simulink model "Case3_IEEE39_UGFLandGFM_2022b"  (R2022b)
settings: Solver=VariableStepAuto  StartTime=0.0  StopTime=30  RelTol=1e-3
InitFcn:
  | IEEE39data_UGFLandGFM;
undefined symbols (not defined in the file): Fref, IBR, line, Sbase, SG, UGFML, Vbase
libraries: spsThreePhaseVIMeasurementLib x66, spsThreePhasePISectionLineLib x35, spsPLL3phLib x25, spsControlledVoltageSourceLib x21, spsThreePhaseParallelRLCLoadLib x21, powerlib_extras x20, spsGroundLib x20, spsMeanLib x20, spsRMSLib x15, spsabctodq0Lib x11, spsThreePhaseSeriesRLCBranchLib x10, slpidlib x10
(part 4 of 5)

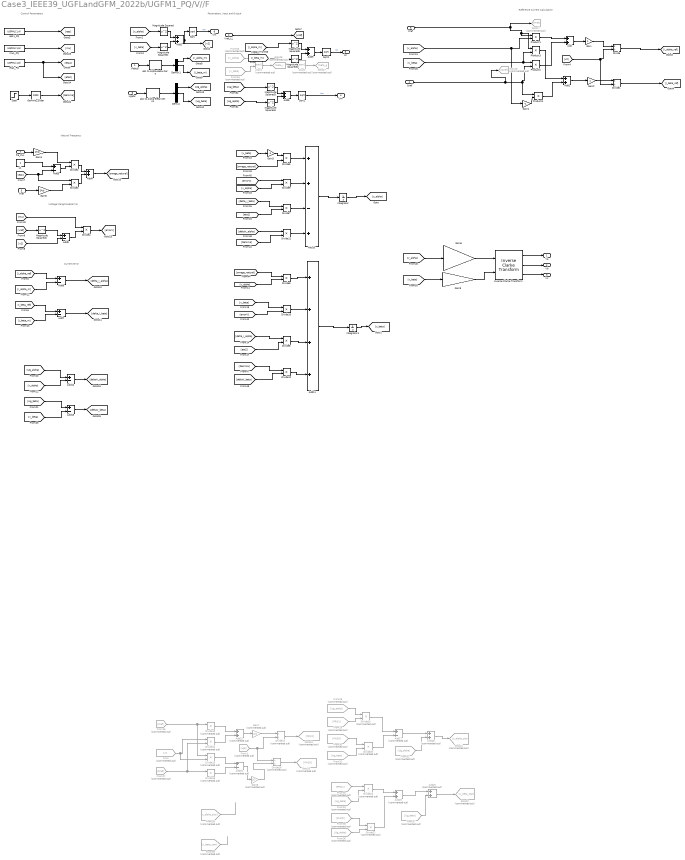
== system Case3_IEEE39_UGFLandGFM_2022b/UGFM1_PQ/V//F ==
  note: Natural Frequency
  note: Voltage Mangnitude Errror
  note: Current Error
  note: Control Parameters
  note: Parameters, Input and Output
  note: Reference Current Calculation
  iFabcb : Inport
  Vref_LL : Inport  Port=2
  Fref : Inport  Port=3
  Qref : Inport  Port=4
  Pref : Inport  Port=5
  Ugabc : Inport  Port=6
  fre_PLL : Inport  Port=7
  Add{,1..2,4,8..9} (6 alike) : Sum
  Add10 : Sum  Inputs=++-+
  Add11 : Sum  Inputs=++++
  Add{3,5..7,12..13} (6 alike) : Sum  Inputs=+-
  Add{15,18..20} (4 alike) : Sum  Commented=on
  Add16 : Sum  Commented=on  Inputs=+-
  Add17 : Sum  Commented=on  Inputs=+-
  Atan1 : Trigonometry  Commented=on  Operator=atan2
  Atan2 : Trigonometry  Commented=on  Operator=atan2
  Demux : Demux  Outputs=3
  Demux1 : Demux  Outputs=3
  Divide : Product  Inputs=*/
  Divide1 : Product  Inputs=*/
  Divide{2..12} (11 alike) : Product  Inputs=**
  Divide{13..16,19..22} (8 alike) : Product  Commented=on  Inputs=**
  Divide17 : Product  Commented=on  Inputs=*/
  Divide18 : Product  Commented=on  Inputs=/*
  From : From  Commented=on  GotoTag=X
  From1 : From  Commented=on  GotoTag=ug2
  From26 : From  Commented=on  GotoTag=Pref
  From27 : From  Commented=on  GotoTag=Qref
  From28 : From  Commented=on  GotoTag=Ug_alpha
  From29 : From  Commented=on  GotoTag=PRQX
  From30 : From  Commented=on  GotoTag=PXQR
  From31 : From  Commented=on  GotoTag=Ug_beta
  From32 : From  Commented=on  GotoTag=Ug_alpha
  From33 : From  Commented=on  GotoTag=PRQX
  From34 : From  Commented=on  GotoTag=Ug_beta
  From35 : From  Commented=on  GotoTag=PXQR
  From36 : From  Commented=on  GotoTag=Ug_alpha
  From37 : From  Commented=on  GotoTag=Ug_beta
  From38 : From  Commented=on  GotoTag=v_alpha_star
  From39 : From  Commented=on  GotoTag=v_beta_star
  From53 : From  Commented=on  GotoTag=v_alpha
  From54 : From  Commented=on  GotoTag=v_beta
  Gain : Gain
  Gain1 : Gain  Gain=-1
  Gain2 : Gain
  Gain3 : Gain  Gain=-1
  Gain4 : Gain  Gain=2*pi
  Gain5 : Gain  Gain=2*pi
  Gain6 : Gain  Gain=Vbase/sqrt(3)*sqrt(2)
  Gain7 : Gain  Commented=on  Gain=2/3
  Gain8 : Gain  Commented=on  Gain=2/3
  Gain9 : Gain  Gain=Vbase/sqrt(3)*sqrt(2)
  Gamma_Slider : simulink/Math Operations/Slider Gain  gain=1000  low=0  high=1000
  Goto17 : Goto  Commented=on  GotoTag=Pref
  Goto18 : Goto  Commented=on  GotoTag=Qref
  Goto19 : Goto  Commented=on  GotoTag=PRQX
  Goto20 : Goto  Commented=on  GotoTag=PXQR
  Goto21 : Goto  Commented=on  GotoTag=v_alpha_star
  Goto22 : Goto  Commented=on  GotoTag=v_beta_star
  Goto27 : Goto  Commented=on  GotoTag=theta_g  TagVisibility=global
  Goto28 : Goto  Commented=on  GotoTag=theta_i  TagVisibility=global
  Integrator : Integrator  InitialCondition=1  LimitOutput=on  UpperSaturationLimit=2  LowerSaturationLimit=-2  ZeroCross=off
  Integrator1 : Integrator  InitialCondition=0.0001  LimitOutput=on  UpperSaturationLimit=2  LowerSaturationLimit=-2  ZeroCross=off
  Inverse Clarke Transform : mcbcontrolslib/Inverse Clarke Transform  PhaseInput=Two inputs  EnPowerInv=off
      settings: LibrarySourceBlock=mcblib/Controls/Math Transforms/Inverse Clarke Transform
  Magnitude Squared{,1..6} (7 alike) : Math  Operator=square
  Product{1..4} (4 alike) : Product
  Sqrt : Sqrt
  Sqrt1 : Sqrt
  Sqrt2 : Sqrt
  Step : Step  Time=0.1  Before=1  After=0  SampleTime=0
  abc to Alpha-Beta-Zero : spsabctoAlphaBetaZeroLib/abc to Alpha-Beta-Zero
  abc to Alpha-Beta-Zero1 : spsabctoAlphaBetaZeroLib/abc to Alpha-Beta-Zero
  eps1_PQ : Constant  Value=UGFML(1,4)
  eta1_PQ : Constant  Value=UGFML(1,6)
  mu1_PQ : Constant  Value=UGFML(1,5)
  u1 : Constant
  Va : Outport
  Vb : Outport  Port=2
  Vc : Outport  Port=3
  Um : Outport  Port=4
  Im : Outport  Port=5
  Vm : Outport  Port=6
  wires:
  iFabcb/1 -> abc to Alpha-Beta-Zero/1
  Inverse Clarke Transform/1 -> Va/1
  Inverse Clarke Transform/2 -> Vb/1
  Inverse Clarke Transform/3 -> Vc/1
  abc to Alpha-Beta-Zero/1 -> Demux1/1
  Integrator1/1 -> [v_beta]
  Pref/1 -> Product3/1, Product1/1, Goto17/1
  [v_alpha] -> Gain1/1, Product1/2
  [v_beta] -> Product3/2, Product2/1
  Qref/1 -> Goto18/1, Product2/2, Product4/1
  Product1/1 -> Add/1
  Product2/1 -> Add/2
  Gain1/1 -> Product4/2
  Product3/1 -> Add1/1
  Product4/1 -> Add1/2
  Add/1 -> Gain/1
  Add1/1 -> Gain2/1
  [v_alpha] -> Magnitude Squared/1
  [v_beta] -> Magnitude Squared1/1
  Magnitude Squared/1 -> Add2/1
  Magnitude Squared1/1 -> Add2/2
  Gain/1 -> Divide/1
  [v2] -> Divide/2, Divide1/2
  Gain2/1 -> Divide1/1
  Divide/1 -> [i_alpha_ref]
  Divide1/1 -> [i_beta_ref]
  u1/1 -> Add3/1
  [eps] -> Divide3/1, Add3/2
  Add3/1 -> Divide2/2
  Fref/1 -> Gain5/1
  Divide2/1 -> Add4/1
  Divide3/1 -> Add4/2
  [v2] -> Add5/2
  Magnitude Squared2/1 -> Add5/1
  Add5/1 -> Divide4/2
  [errorV] -> Divide10/2
  [omega_natural] -> Divide5/2
  [v_beta] -> Gain3/1
  Gain3/1 -> Divide5/1
  [v_alpha] -> Divide6/2
  [i_alpha_ref] -> Add6/1
  [i_alpha_m] -> Add6/2
  [i_beta_ref] -> Add7/1
  Demux1/1 -> [i_alpha_m]
  Demux1/2 -> [i_beta_m]
  [i_beta_m] -> Add7/2
  Add6/1 -> [delta_i_alpha]
  Add7/1 -> [delta_i_beta]
  [delta_i_beta] -> Divide7/1
  [eta1] -> Divide7/2
  Divide7/1 -> Add10/3
  [delta_i_alpha] -> Divide8/1
  [eta2] -> Divide8/2
  Divide8/1 -> Add11/3
  Add10/1 -> Integrator/1
  Add11/1 -> Integrator1/1
  Gain5/1 -> Divide3/2
  Vref_LL/1 -> [vref]
  [vref] -> Magnitude Squared2/1
  [v_alpha] -> Divide9/2
  [v_beta] -> Divide10/1
  Divide5/1 -> Add10/1
  Divide9/1 -> Add10/2
  Divide6/1 -> Add11/1
  Divide10/1 -> Add11/2
  Ugabc/1 -> abc to Alpha-Beta-Zero1/1
  abc to Alpha-Beta-Zero1/1 -> Demux/1
  From38/1 -> ?
  [v_alpha] -> Add12/2
  From39/1 -> ?
  [v_beta] -> Add13/2
  Add12/1 -> [deltaV_alpha]
  Add13/1 -> [deltaV_beta]
  Divide11/1 -> Add10/4
  Divide12/1 -> Add11/4
  eta1_PQ/1 -> [eta2], [eta1]
  Gain4/1 -> Divide2/1
  Demux/1 -> [Ug_alpha]
  Demux/2 -> [Ug_beta]
  From26/1 -> Divide15/1, Divide13/1
  From/1 -> Divide15/2, Divide14/1
  From27/1 -> Divide16/1, Divide14/2
  Divide13/1 -> Add15/1
  Divide14/1 -> Add15/2
  Divide15/1 -> Add16/1
  Divide16/1 -> Add16/2
  Gain7/1 -> Divide17/1
  Gain8/1 -> Divide18/2
  From1/1 -> Divide18/1, Divide17/2
  Add15/1 -> Gain7/1
  Add16/1 -> Gain8/1
  Divide17/1 -> Goto19/1
  Divide18/1 -> Goto20/1
  From28/1 -> Divide19/1
  From29/1 -> Divide19/2
  From30/1 -> Divide20/1
  From31/1 -> Divide20/2
  Divide19/1 -> Add17/1
  Divide20/1 -> Add17/2
  Add17/1 -> Add18/1
  From32/1 -> Add18/2
  From33/1 -> Divide21/1
  From34/1 -> Divide21/2
  From35/1 -> Divide22/1
  From36/1 -> Divide22/2
  Divide21/1 -> Add19/1
  Divide22/1 -> Add19/2
  Add19/1 -> Add20/1
  From37/1 -> Add20/2
  Add18/1 -> Goto21/1
  Add20/1 -> Goto22/1
  [Ug_alpha] -> Add12/1
  [Ug_beta] -> Add13/1
  [mu] -> Divide4/1
  eps1_PQ/1 -> [eps]
  Step/1 -> Gamma_Slider/1
  Gamma_Slider/1 -> [Gamma]
  [Gamma] -> Divide11/2
  Divide4/1 -> [errorV]
  Add4/1 -> [omega_natural]
  [omega_natural] -> Divide6/1
  [errorV] -> Divide9/1
  Integrator/1 -> [v_alpha]
  [v_alpha] -> Gain6/1
  [Gamma] -> Divide12/1
  [deltaV_alpha] -> Divide11/1
  [deltaV_beta] -> Divide12/2
  [v_beta] -> Gain9/1
  Gain6/1 -> Inverse Clarke Transform/1
  Gain9/1 -> Inverse Clarke Transform/2
  Atan2/1 -> Goto27/1
  From53/1 -> Atan1/1
  From54/1 -> Atan1/2
  Atan1/1 -> Goto28/1
  fre_PLL/1 -> Gain4/1
  Sqrt/1 -> Vm/1  "Vm"
  Add2/1 -> [v2], Sqrt/1
  Magnitude Squared3/1 -> Add8/1
  [Ug_beta] -> Magnitude Squared3/1
  Magnitude Squared4/1 -> Add8/2
  [Ug_alpha] -> Magnitude Squared4/1
  Add8/1 -> Sqrt1/1
  Sqrt1/1 -> Um/1  "Um"
  Magnitude Squared5/1 -> Add9/1
  Sqrt2/1 -> Im/1  "Im"
  [i_beta_m] -> Magnitude Squared6/1
  Add9/1 -> Sqrt2/1
  [i_alpha_m] -> Magnitude Squared5/1
  Magnitude Squared6/1 -> Add9/2
  mu1_PQ/1 -> [mu]

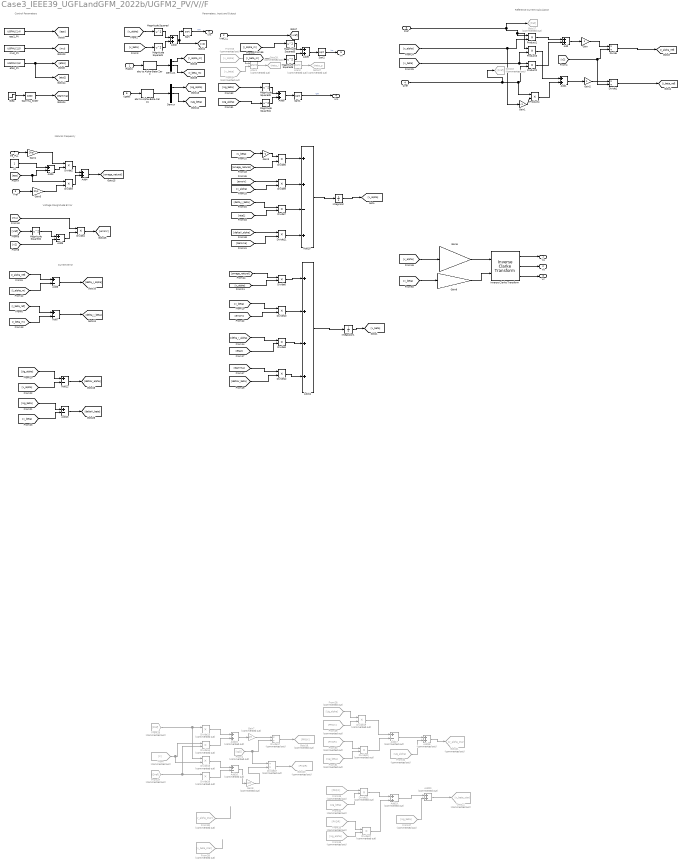
== system Case3_IEEE39_UGFLandGFM_2022b/UGFM2_PV/V//F ==
  note: Natural Frequency
  note: Voltage Mangnitude Errror
  note: Current Error
  note: Control Parameters
  note: Parameters, Input and Output
  note: Reference Current Calculation
  iFabcb : Inport
  Vref_LL : Inport  Port=2
  Fref : Inport  Port=3
  Qref : Inport  Port=4
  Pref : Inport  Port=5
  Ugabc : Inport  Port=6
  fre_PLL : Inport  Port=7
  Add{,1..2,4,8..9} (6 alike) : Sum
  Add10 : Sum  Inputs=++-+
  Add11 : Sum  Inputs=++++
  Add{3,5..7,12..13} (6 alike) : Sum  Inputs=+-
  Add{15,18..20} (4 alike) : Sum  Commented=on
  Add16 : Sum  Commented=on  Inputs=+-
  Add17 : Sum  Commented=on  Inputs=+-
  Atan1 : Trigonometry  Commented=on  Operator=atan2
  Atan2 : Trigonometry  Commented=on  Operator=atan2
  Demux : Demux  Outputs=3
  Demux1 : Demux  Outputs=3
  Divide : Product  Inputs=*/
  Divide1 : Product  Inputs=*/
  Divide{2..12} (11 alike) : Product  Inputs=**
  Divide{13..16,19..22} (8 alike) : Product  Commented=on  Inputs=**
  Divide17 : Product  Commented=on  Inputs=*/
  Divide18 : Product  Commented=on  Inputs=/*
  From : From  Commented=on  GotoTag=X
  From1 : From  Commented=on  GotoTag=ug2
  From26 : From  Commented=on  GotoTag=Pref
  From27 : From  Commented=on  GotoTag=Qref
  From28 : From  Commented=on  GotoTag=Ug_alpha
  From29 : From  Commented=on  GotoTag=PRQX
  From30 : From  Commented=on  GotoTag=PXQR
  From31 : From  Commented=on  GotoTag=Ug_beta
  From32 : From  Commented=on  GotoTag=Ug_alpha
  From33 : From  Commented=on  GotoTag=PRQX
  From34 : From  Commented=on  GotoTag=Ug_beta
  From35 : From  Commented=on  GotoTag=PXQR
  From36 : From  Commented=on  GotoTag=Ug_alpha
  From37 : From  Commented=on  GotoTag=Ug_beta
  From38 : From  Commented=on  GotoTag=v_alpha_star
  From39 : From  Commented=on  GotoTag=v_beta_star
  From53 : From  Commented=on  GotoTag=v_alpha
  From54 : From  Commented=on  GotoTag=v_beta
  Gain : Gain
  Gain1 : Gain  Gain=-1
  Gain2 : Gain
  Gain3 : Gain  Gain=-1
  Gain4 : Gain  Gain=2*pi
  Gain5 : Gain  Gain=2*pi
  Gain6 : Gain  Gain=Vbase/sqrt(3)*sqrt(2)
  Gain7 : Gain  Commented=on  Gain=2/3
  Gain8 : Gain  Commented=on  Gain=2/3
  Gain9 : Gain  Gain=Vbase/sqrt(3)*sqrt(2)
  Gamma_Slider : simulink/Math Operations/Slider Gain  gain=1000  low=0  high=1000
  Goto17 : Goto  Commented=on  GotoTag=Pref
  Goto18 : Goto  Commented=on  GotoTag=Qref
  Goto19 : Goto  Commented=on  GotoTag=PRQX
  Goto20 : Goto  Commented=on  GotoTag=PXQR
  Goto21 : Goto  Commented=on  GotoTag=v_alpha_star
  Goto22 : Goto  Commented=on  GotoTag=v_beta_star
  Goto27 : Goto  Commented=on  GotoTag=theta_g  TagVisibility=global
  Goto28 : Goto  Commented=on  GotoTag=theta_i  TagVisibility=global
  Integrator : Integrator  InitialCondition=1  LimitOutput=on  UpperSaturationLimit=2  LowerSaturationLimit=-2  ZeroCross=off
  Integrator1 : Integrator  InitialCondition=0.0001  LimitOutput=on  UpperSaturationLimit=2  LowerSaturationLimit=-2  ZeroCross=off
  Inverse Clarke Transform : mcbcontrolslib/Inverse Clarke Transform  PhaseInput=Two inputs  EnPowerInv=off
      settings: LibrarySourceBlock=mcblib/Controls/Math Transforms/Inverse Clarke Transform
  Magnitude Squared{,1..6} (7 alike) : Math  Operator=square
  Product{1..4} (4 alike) : Product
  Sqrt : Sqrt
  Sqrt1 : Sqrt
  Sqrt2 : Sqrt
  Step : Step  Time=0.1  Before=1  After=0  SampleTime=0
  abc to Alpha-Beta-Zero : spsabctoAlphaBetaZeroLib/abc to Alpha-Beta-Zero
  abc to Alpha-Beta-Zero1 : spsabctoAlphaBetaZeroLib/abc to Alpha-Beta-Zero
  eps2_PV : Constant  Value=UGFML(2,4)
  eta2_PV : Constant  Value=UGFML(2,6)
  mu2_PV : Constant  Value=UGFML(2,5)
  u1 : Constant
  Va : Outport
  Vb : Outport  Port=2
  Vc : Outport  Port=3
  Um : Outport  Port=4
  Im : Outport  Port=5
  Vm : Outport  Port=6
  wires:
  iFabcb/1 -> abc to Alpha-Beta-Zero/1
  Inverse Clarke Transform/1 -> Va/1
  Inverse Clarke Transform/2 -> Vb/1
  Inverse Clarke Transform/3 -> Vc/1
  abc to Alpha-Beta-Zero/1 -> Demux1/1
  Integrator1/1 -> [v_beta]
  Pref/1 -> Product3/1, Product1/1, Goto17/1
  [v_alpha] -> Gain1/1, Product1/2
  [v_beta] -> Product3/2, Product2/1
  Qref/1 -> Goto18/1, Product2/2, Product4/1
  Product1/1 -> Add/1
  Product2/1 -> Add/2
  Gain1/1 -> Product4/2
  Product3/1 -> Add1/1
  Product4/1 -> Add1/2
  Add/1 -> Gain/1
  Add1/1 -> Gain2/1
  [v_alpha] -> Magnitude Squared/1
  [v_beta] -> Magnitude Squared1/1
  Magnitude Squared/1 -> Add2/1
  Magnitude Squared1/1 -> Add2/2
  Gain/1 -> Divide/1
  [v2] -> Divide/2, Divide1/2
  Gain2/1 -> Divide1/1
  Divide/1 -> [i_alpha_ref]
  Divide1/1 -> [i_beta_ref]
  u1/1 -> Add3/1
  [eps] -> Divide3/1, Add3/2
  Add3/1 -> Divide2/2
  Fref/1 -> Gain5/1
  Divide2/1 -> Add4/1
  Divide3/1 -> Add4/2
  [v2] -> Add5/2
  Magnitude Squared2/1 -> Add5/1
  Add5/1 -> Divide4/2
  [errorV] -> Divide10/2
  [omega_natural] -> Divide5/2
  [v_beta] -> Gain3/1
  Gain3/1 -> Divide5/1
  [v_alpha] -> Divide6/2
  [i_alpha_ref] -> Add6/1
  [i_alpha_m] -> Add6/2
  [i_beta_ref] -> Add7/1
  Demux1/1 -> [i_alpha_m]
  Demux1/2 -> [i_beta_m]
  [i_beta_m] -> Add7/2
  Add6/1 -> [delta_i_alpha]
  Add7/1 -> [delta_i_beta]
  [delta_i_beta] -> Divide7/1
  [eta1] -> Divide7/2
  Divide7/1 -> Add10/3
  [delta_i_alpha] -> Divide8/1
  [eta2] -> Divide8/2
  Divide8/1 -> Add11/3
  Add10/1 -> Integrator/1
  Add11/1 -> Integrator1/1
  Gain5/1 -> Divide3/2
  Vref_LL/1 -> [vref]
  [vref] -> Magnitude Squared2/1
  [v_alpha] -> Divide9/2
  [v_beta] -> Divide10/1
  Divide5/1 -> Add10/1
  Divide9/1 -> Add10/2
  Divide6/1 -> Add11/1
  Divide10/1 -> Add11/2
  Ugabc/1 -> abc to Alpha-Beta-Zero1/1
  abc to Alpha-Beta-Zero1/1 -> Demux/1
  From38/1 -> ?
  [v_alpha] -> Add12/2
  From39/1 -> ?
  [v_beta] -> Add13/2
  Add12/1 -> [deltaV_alpha]
  Add13/1 -> [deltaV_beta]
  Divide11/1 -> Add10/4
  Divide12/1 -> Add11/4
  eta2_PV/1 -> [eta2], [eta1]
  Gain4/1 -> Divide2/1
  Demux/1 -> [Ug_alpha]
  Demux/2 -> [Ug_beta]
  From26/1 -> Divide15/1, Divide13/1
  From/1 -> Divide15/2, Divide14/1
  From27/1 -> Divide16/1, Divide14/2
  Divide13/1 -> Add15/1
  Divide14/1 -> Add15/2
  Divide15/1 -> Add16/1
  Divide16/1 -> Add16/2
  Gain7/1 -> Divide17/1
  Gain8/1 -> Divide18/2
  From1/1 -> Divide18/1, Divide17/2
  Add15/1 -> Gain7/1
  Add16/1 -> Gain8/1
  Divide17/1 -> Goto19/1
  Divide18/1 -> Goto20/1
  From28/1 -> Divide19/1
  From29/1 -> Divide19/2
  From30/1 -> Divide20/1
  From31/1 -> Divide20/2
  Divide19/1 -> Add17/1
  Divide20/1 -> Add17/2
  Add17/1 -> Add18/1
  From32/1 -> Add18/2
  From33/1 -> Divide21/1
  From34/1 -> Divide21/2
  From35/1 -> Divide22/1
  From36/1 -> Divide22/2
  Divide21/1 -> Add19/1
  Divide22/1 -> Add19/2
  Add19/1 -> Add20/1
  From37/1 -> Add20/2
  Add18/1 -> Goto21/1
  Add20/1 -> Goto22/1
  [Ug_alpha] -> Add12/1
  [Ug_beta] -> Add13/1
  mu2_PV/1 -> [mu]
  [mu] -> Divide4/1
  eps2_PV/1 -> [eps]
  Step/1 -> Gamma_Slider/1
  Gamma_Slider/1 -> [Gamma]
  [Gamma] -> Divide11/2
  Divide4/1 -> [errorV]
  Add4/1 -> [omega_natural]
  [omega_natural] -> Divide6/1
  [errorV] -> Divide9/1
  Integrator/1 -> [v_alpha]
  [v_alpha] -> Gain6/1
  [Gamma] -> Divide12/1
  [deltaV_alpha] -> Divide11/1
  [deltaV_beta] -> Divide12/2
  [v_beta] -> Gain9/1
  Gain6/1 -> Inverse Clarke Transform/1
  Gain9/1 -> Inverse Clarke Transform/2
  Atan2/1 -> Goto27/1
  From53/1 -> Atan1/1
  From54/1 -> Atan1/2
  Atan1/1 -> Goto28/1
  fre_PLL/1 -> Gain4/1
  Sqrt/1 -> Vm/1  "Vm"
  Add2/1 -> [v2], Sqrt/1
  Magnitude Squared3/1 -> Add8/1
  [Ug_beta] -> Magnitude Squared3/1
  Magnitude Squared4/1 -> Add8/2
  [Ug_alpha] -> Magnitude Squared4/1
  Add8/1 -> Sqrt1/1
  Sqrt1/1 -> Um/1  "Um"
  Magnitude Squared5/1 -> Add9/1
  Sqrt2/1 -> Im/1  "Im"
  [i_beta_m] -> Magnitude Squared6/1
  Add9/1 -> Sqrt2/1
  [i_alpha_m] -> Magnitude Squared5/1
  Magnitude Squared6/1 -> Add9/2

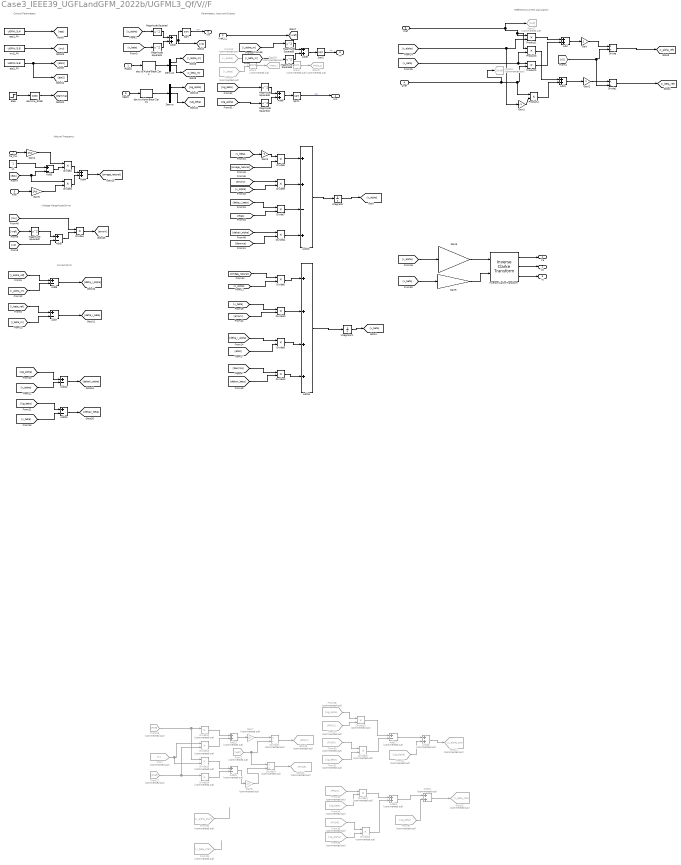
== system Case3_IEEE39_UGFLandGFM_2022b/UGFML3_Qf/V//F ==
  note: Natural Frequency
  note: Voltage Mangnitude Errror
  note: Current Error
  note: Control Parameters
  note: Parameters, Input and Output
  note: Reference Current Calculation
  iFabcb : Inport
  Vref_LL : Inport  Port=2
  Fref : Inport  Port=3
  Qref : Inport  Port=4
  Pref : Inport  Port=5
  Ugabc : Inport  Port=6
  fre_PLL : Inport  Port=7
  Add{,1..2,4,8..9} (6 alike) : Sum
  Add10 : Sum  Inputs=++-+
  Add11 : Sum  Inputs=++++
  Add{3,5..7,12..13} (6 alike) : Sum  Inputs=+-
  Add{15,18..20} (4 alike) : Sum  Commented=on
  Add16 : Sum  Commented=on  Inputs=+-
  Add17 : Sum  Commented=on  Inputs=+-
  Atan1 : Trigonometry  Commented=on  Operator=atan2
  Atan2 : Trigonometry  Commented=on  Operator=atan2
  Demux : Demux  Outputs=3
  Demux1 : Demux  Outputs=3
  Divide : Product  Inputs=*/
  Divide1 : Product  Inputs=*/
  Divide{2..12} (11 alike) : Product  Inputs=**
  Divide{13..16,19..22} (8 alike) : Product  Commented=on  Inputs=**
  Divide17 : Product  Commented=on  Inputs=*/
  Divide18 : Product  Commented=on  Inputs=/*
  From : From  Commented=on  GotoTag=X
  From1 : From  Commented=on  GotoTag=ug2
  From26 : From  Commented=on  GotoTag=Pref
  From27 : From  Commented=on  GotoTag=Qref
  From28 : From  Commented=on  GotoTag=Ug_alpha
  From29 : From  Commented=on  GotoTag=PRQX
  From30 : From  Commented=on  GotoTag=PXQR
  From31 : From  Commented=on  GotoTag=Ug_beta
  From32 : From  Commented=on  GotoTag=Ug_alpha
  From33 : From  Commented=on  GotoTag=PRQX
  From34 : From  Commented=on  GotoTag=Ug_beta
  From35 : From  Commented=on  GotoTag=PXQR
  From36 : From  Commented=on  GotoTag=Ug_alpha
  From37 : From  Commented=on  GotoTag=Ug_beta
  From38 : From  Commented=on  GotoTag=v_alpha_star
  From39 : From  Commented=on  GotoTag=v_beta_star
  From53 : From  Commented=on  GotoTag=v_alpha
  From54 : From  Commented=on  GotoTag=v_beta
  Gain : Gain
  Gain1 : Gain  Gain=-1
  Gain2 : Gain
  Gain3 : Gain  Gain=-1
  Gain4 : Gain  Gain=2*pi
  Gain5 : Gain  Gain=2*pi
  Gain6 : Gain  Gain=Vbase/sqrt(3)*sqrt(2)
  Gain7 : Gain  Commented=on  Gain=2/3
  Gain8 : Gain  Commented=on  Gain=2/3
  Gain9 : Gain  Gain=Vbase/sqrt(3)*sqrt(2)
  Gamma_Slider : simulink/Math Operations/Slider Gain  gain=1000  low=0  high=1000
  Goto17 : Goto  Commented=on  GotoTag=Pref
  Goto18 : Goto  Commented=on  GotoTag=Qref
  Goto19 : Goto  Commented=on  GotoTag=PRQX
  Goto20 : Goto  Commented=on  GotoTag=PXQR
  Goto21 : Goto  Commented=on  GotoTag=v_alpha_star
  Goto22 : Goto  Commented=on  GotoTag=v_beta_star
  Goto27 : Goto  Commented=on  GotoTag=theta_g  TagVisibility=global
  Goto28 : Goto  Commented=on  GotoTag=theta_i  TagVisibility=global
  Integrator : Integrator  InitialCondition=1  LimitOutput=on  UpperSaturationLimit=2  LowerSaturationLimit=-2  ZeroCross=off
  Integrator1 : Integrator  InitialCondition=0.0001  LimitOutput=on  UpperSaturationLimit=2  LowerSaturationLimit=-2  ZeroCross=off
  Inverse Clarke Transform : mcbcontrolslib/Inverse Clarke Transform  PhaseInput=Two inputs  EnPowerInv=off
      settings: LibrarySourceBlock=mcblib/Controls/Math Transforms/Inverse Clarke Transform
  Magnitude Squared{,1..6} (7 alike) : Math  Operator=square
  Product{1..4} (4 alike) : Product
  Sqrt : Sqrt
  Sqrt1 : Sqrt
  Sqrt2 : Sqrt
  Step : Step  Time=0.1  Before=1  After=0  SampleTime=0
  abc to Alpha-Beta-Zero : spsabctoAlphaBetaZeroLib/abc to Alpha-Beta-Zero
  abc to Alpha-Beta-Zero1 : spsabctoAlphaBetaZeroLib/abc to Alpha-Beta-Zero
  eps2_PV : Constant  Value=UGFML(3,4)
  eta2_PV : Constant  Value=UGFML(3,6)
  mu2_PV : Constant  Value=UGFML(3,5)
  u1 : Constant
  Va : Outport
  Vb : Outport  Port=2
  Vc : Outport  Port=3
  Um : Outport  Port=4
  Im : Outport  Port=5
  Vm : Outport  Port=6
  wires:
  iFabcb/1 -> abc to Alpha-Beta-Zero/1
  Inverse Clarke Transform/1 -> Va/1
  Inverse Clarke Transform/2 -> Vb/1
  Inverse Clarke Transform/3 -> Vc/1
  abc to Alpha-Beta-Zero/1 -> Demux1/1
  Integrator1/1 -> [v_beta]
  Pref/1 -> Product3/1, Product1/1, Goto17/1
  [v_alpha] -> Gain1/1, Product1/2
  [v_beta] -> Product3/2, Product2/1
  Qref/1 -> Goto18/1, Product2/2, Product4/1
  Product1/1 -> Add/1
  Product2/1 -> Add/2
  Gain1/1 -> Product4/2
  Product3/1 -> Add1/1
  Product4/1 -> Add1/2
  Add/1 -> Gain/1
  Add1/1 -> Gain2/1
  [v_alpha] -> Magnitude Squared/1
  [v_beta] -> Magnitude Squared1/1
  Magnitude Squared/1 -> Add2/1
  Magnitude Squared1/1 -> Add2/2
  Gain/1 -> Divide/1
  [v2] -> Divide/2, Divide1/2
  Gain2/1 -> Divide1/1
  Divide/1 -> [i_alpha_ref]
  Divide1/1 -> [i_beta_ref]
  u1/1 -> Add3/1
  [eps] -> Divide3/1, Add3/2
  Add3/1 -> Divide2/2
  Fref/1 -> Gain5/1
  Divide2/1 -> Add4/1
  Divide3/1 -> Add4/2
  [v2] -> Add5/2
  Magnitude Squared2/1 -> Add5/1
  Add5/1 -> Divide4/2
  [errorV] -> Divide10/2
  [omega_natural] -> Divide5/2
  [v_beta] -> Gain3/1
  Gain3/1 -> Divide5/1
  [v_alpha] -> Divide6/2
  [i_alpha_ref] -> Add6/1
  [i_alpha_m] -> Add6/2
  [i_beta_ref] -> Add7/1
  Demux1/1 -> [i_alpha_m]
  Demux1/2 -> [i_beta_m]
  [i_beta_m] -> Add7/2
  Add6/1 -> [delta_i_alpha]
  Add7/1 -> [delta_i_beta]
  [delta_i_beta] -> Divide7/1
  [eta1] -> Divide7/2
  Divide7/1 -> Add10/3
  [delta_i_alpha] -> Divide8/1
  [eta2] -> Divide8/2
  Divide8/1 -> Add11/3
  Add10/1 -> Integrator/1
  Add11/1 -> Integrator1/1
  Gain5/1 -> Divide3/2
  Vref_LL/1 -> [vref]
  [vref] -> Magnitude Squared2/1
  [v_alpha] -> Divide9/2
  [v_beta] -> Divide10/1
  Divide5/1 -> Add10/1
  Divide9/1 -> Add10/2
  Divide6/1 -> Add11/1
  Divide10/1 -> Add11/2
  Ugabc/1 -> abc to Alpha-Beta-Zero1/1
  abc to Alpha-Beta-Zero1/1 -> Demux/1
  From38/1 -> ?
  [v_alpha] -> Add12/2
  From39/1 -> ?
  [v_beta] -> Add13/2
  Add12/1 -> [deltaV_alpha]
  Add13/1 -> [deltaV_beta]
  Divide11/1 -> Add10/4
  Divide12/1 -> Add11/4
  Gain4/1 -> Divide2/1
  Demux/1 -> [Ug_alpha]
  Demux/2 -> [Ug_beta]
  From26/1 -> Divide15/1, Divide13/1
  From/1 -> Divide15/2, Divide14/1
  From27/1 -> Divide16/1, Divide14/2
  Divide13/1 -> Add15/1
  Divide14/1 -> Add15/2
  Divide15/1 -> Add16/1
  Divide16/1 -> Add16/2
  Gain7/1 -> Divide17/1
  Gain8/1 -> Divide18/2
  From1/1 -> Divide18/1, Divide17/2
  Add15/1 -> Gain7/1
  Add16/1 -> Gain8/1
  Divide17/1 -> Goto19/1
  Divide18/1 -> Goto20/1
  From28/1 -> Divide19/1
  From29/1 -> Divide19/2
  From30/1 -> Divide20/1
  From31/1 -> Divide20/2
  Divide19/1 -> Add17/1
  Divide20/1 -> Add17/2
  Add17/1 -> Add18/1
  From32/1 -> Add18/2
  From33/1 -> Divide21/1
  From34/1 -> Divide21/2
  From35/1 -> Divide22/1
  From36/1 -> Divide22/2
  Divide21/1 -> Add19/1
  Divide22/1 -> Add19/2
  Add19/1 -> Add20/1
  From37/1 -> Add20/2
  Add18/1 -> Goto21/1
  Add20/1 -> Goto22/1
  [Ug_alpha] -> Add12/1
  [Ug_beta] -> Add13/1
  [mu] -> Divide4/1
  Step/1 -> Gamma_Slider/1
  Gamma_Slider/1 -> [Gamma]
  [Gamma] -> Divide11/2
  Divide4/1 -> [errorV]
  Add4/1 -> [omega_natural]
  [omega_natural] -> Divide6/1
  [errorV] -> Divide9/1
  Integrator/1 -> [v_alpha]
  [v_alpha] -> Gain6/1
  [Gamma] -> Divide12/1
  [deltaV_alpha] -> Divide11/1
  [deltaV_beta] -> Divide12/2
  [v_beta] -> Gain9/1
  Gain6/1 -> Inverse Clarke Transform/1
  Gain9/1 -> Inverse Clarke Transform/2
  Atan2/1 -> Goto27/1
  From53/1 -> Atan1/1
  From54/1 -> Atan1/2
  Atan1/1 -> Goto28/1
  fre_PLL/1 -> Gain4/1
  Sqrt/1 -> Vm/1  "Vm"
  Add2/1 -> [v2], Sqrt/1
  Magnitude Squared3/1 -> Add8/1
  [Ug_beta] -> Magnitude Squared3/1
  Magnitude Squared4/1 -> Add8/2
  [Ug_alpha] -> Magnitude Squared4/1
  Add8/1 -> Sqrt1/1
  Sqrt1/1 -> Um/1  "Um"
  Magnitude Squared5/1 -> Add9/1
  Sqrt2/1 -> Im/1  "Im"
  [i_beta_m] -> Magnitude Squared6/1
  Add9/1 -> Sqrt2/1
  [i_alpha_m] -> Magnitude Squared5/1
  Magnitude Squared6/1 -> Add9/2
  eps2_PV/1 -> [eps]
  mu2_PV/1 -> [mu]
  eta2_PV/1 -> [eta2], [eta1]

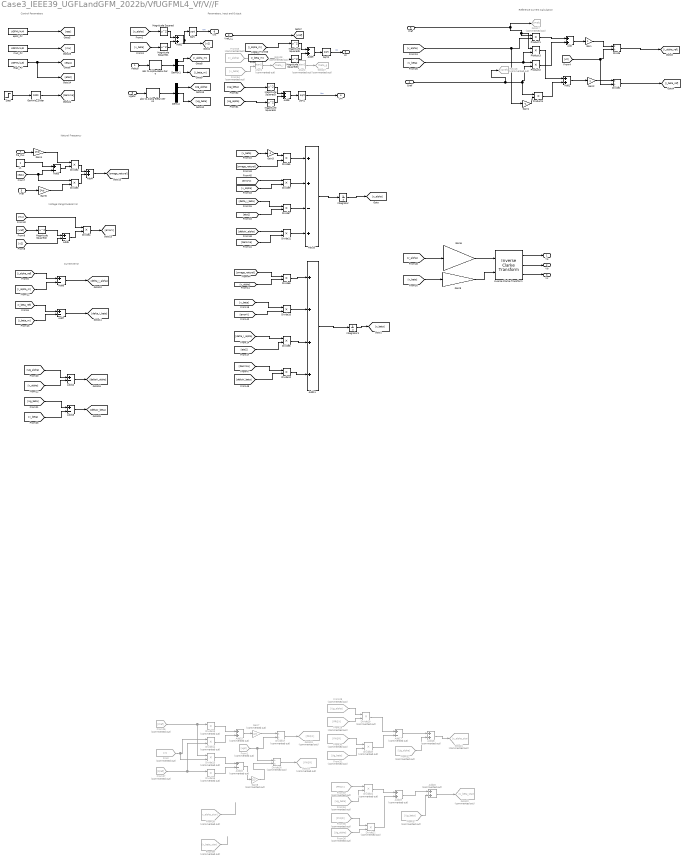
== system Case3_IEEE39_UGFLandGFM_2022b/VfUGFML4_Vf/V//F ==
  note: Natural Frequency
  note: Voltage Mangnitude Errror
  note: Current Error
  note: Control Parameters
  note: Parameters, Input and Output
  note: Reference Current Calculation
  iFabcb : Inport
  Vref_LL : Inport  Port=2
  Fref : Inport  Port=3
  Qref : Inport  Port=4
  Pref : Inport  Port=5
  Ugabc : Inport  Port=6
  fre_PLL : Inport  Port=7
  Add{,1..2,4,8..9} (6 alike) : Sum
  Add10 : Sum  Inputs=++-+
  Add11 : Sum  Inputs=++++
  Add{3,5..7,12..13} (6 alike) : Sum  Inputs=+-
  Add{15,18..20} (4 alike) : Sum  Commented=on
  Add16 : Sum  Commented=on  Inputs=+-
  Add17 : Sum  Commented=on  Inputs=+-
  Atan1 : Trigonometry  Commented=on  Operator=atan2
  Atan2 : Trigonometry  Commented=on  Operator=atan2
  Demux : Demux  Outputs=3
  Demux1 : Demux  Outputs=3
  Divide : Product  Inputs=*/
  Divide1 : Product  Inputs=*/
  Divide{2..12} (11 alike) : Product  Inputs=**
  Divide{13..16,19..22} (8 alike) : Product  Commented=on  Inputs=**
  Divide17 : Product  Commented=on  Inputs=*/
  Divide18 : Product  Commented=on  Inputs=/*
  From : From  Commented=on  GotoTag=X
  From1 : From  Commented=on  GotoTag=ug2
  From26 : From  Commented=on  GotoTag=Pref
  From27 : From  Commented=on  GotoTag=Qref
  From28 : From  Commented=on  GotoTag=Ug_alpha
  From29 : From  Commented=on  GotoTag=PRQX
  From30 : From  Commented=on  GotoTag=PXQR
  From31 : From  Commented=on  GotoTag=Ug_beta
  From32 : From  Commented=on  GotoTag=Ug_alpha
  From33 : From  Commented=on  GotoTag=PRQX
  From34 : From  Commented=on  GotoTag=Ug_beta
  From35 : From  Commented=on  GotoTag=PXQR
  From36 : From  Commented=on  GotoTag=Ug_alpha
  From37 : From  Commented=on  GotoTag=Ug_beta
  From38 : From  Commented=on  GotoTag=v_alpha_star
  From39 : From  Commented=on  GotoTag=v_beta_star
  From53 : From  Commented=on  GotoTag=v_alpha
  From54 : From  Commented=on  GotoTag=v_beta
  Gain : Gain
  Gain1 : Gain  Gain=-1
  Gain2 : Gain
  Gain3 : Gain  Gain=-1
  Gain4 : Gain  Gain=2*pi
  Gain5 : Gain  Gain=2*pi
  Gain6 : Gain  Gain=Vbase/sqrt(3)*sqrt(2)
  Gain7 : Gain  Commented=on  Gain=2/3
  Gain8 : Gain  Commented=on  Gain=2/3
  Gain9 : Gain  Gain=Vbase/sqrt(3)*sqrt(2)
  Gamma_Slider : simulink/Math Operations/Slider Gain  gain=1000  low=0  high=1000
  Goto17 : Goto  Commented=on  GotoTag=Pref
  Goto18 : Goto  Commented=on  GotoTag=Qref
  Goto19 : Goto  Commented=on  GotoTag=PRQX
  Goto20 : Goto  Commented=on  GotoTag=PXQR
  Goto21 : Goto  Commented=on  GotoTag=v_alpha_star
  Goto22 : Goto  Commented=on  GotoTag=v_beta_star
  Goto27 : Goto  Commented=on  GotoTag=theta_g  TagVisibility=global
  Goto28 : Goto  Commented=on  GotoTag=theta_i  TagVisibility=global
  Integrator : Integrator  InitialCondition=1  LimitOutput=on  UpperSaturationLimit=2  LowerSaturationLimit=-2  ZeroCross=off
  Integrator1 : Integrator  InitialCondition=0.0001  LimitOutput=on  UpperSaturationLimit=2  LowerSaturationLimit=-2  ZeroCross=off
  Inverse Clarke Transform : mcbcontrolslib/Inverse Clarke Transform  PhaseInput=Two inputs  EnPowerInv=off
      settings: LibrarySourceBlock=mcblib/Controls/Math Transforms/Inverse Clarke Transform
  Magnitude Squared{,1..6} (7 alike) : Math  Operator=square
  Product{1..4} (4 alike) : Product
  Sqrt : Sqrt
  Sqrt1 : Sqrt
  Sqrt2 : Sqrt
  Step : Step  Time=0.1  Before=1  After=0  SampleTime=0
  abc to Alpha-Beta-Zero : spsabctoAlphaBetaZeroLib/abc to Alpha-Beta-Zero
  abc to Alpha-Beta-Zero1 : spsabctoAlphaBetaZeroLib/abc to Alpha-Beta-Zero
  eps2_PV : Constant  Value=UGFML(4,4)
  eta2_PV : Constant  Value=UGFML(4,6)
  mu2_PV : Constant  Value=UGFML(4,5)
  u1 : Constant
  Va : Outport
  Vb : Outport  Port=2
  Vc : Outport  Port=3
  Um : Outport  Port=4
  Im : Outport  Port=5
  Vm : Outport  Port=6
  wires:
  iFabcb/1 -> abc to Alpha-Beta-Zero/1
  Inverse Clarke Transform/1 -> Va/1
  Inverse Clarke Transform/2 -> Vb/1
  Inverse Clarke Transform/3 -> Vc/1
  abc to Alpha-Beta-Zero/1 -> Demux1/1
  Integrator1/1 -> [v_beta]
  Pref/1 -> Product3/1, Product1/1, Goto17/1
  [v_alpha] -> Gain1/1, Product1/2
  [v_beta] -> Product3/2, Product2/1
  Qref/1 -> Goto18/1, Product2/2, Product4/1
  Product1/1 -> Add/1
  Product2/1 -> Add/2
  Gain1/1 -> Product4/2
  Product3/1 -> Add1/1
  Product4/1 -> Add1/2
  Add/1 -> Gain/1
  Add1/1 -> Gain2/1
  [v_alpha] -> Magnitude Squared/1
  [v_beta] -> Magnitude Squared1/1
  Magnitude Squared/1 -> Add2/1
  Magnitude Squared1/1 -> Add2/2
  Gain/1 -> Divide/1
  [v2] -> Divide/2, Divide1/2
  Gain2/1 -> Divide1/1
  Divide/1 -> [i_alpha_ref]
  Divide1/1 -> [i_beta_ref]
  u1/1 -> Add3/1
  [eps] -> Divide3/1, Add3/2
  Add3/1 -> Divide2/2
  Fref/1 -> Gain5/1
  Divide2/1 -> Add4/1
  Divide3/1 -> Add4/2
  [v2] -> Add5/2
  Magnitude Squared2/1 -> Add5/1
  Add5/1 -> Divide4/2
  [errorV] -> Divide10/2
  [omega_natural] -> Divide5/2
  [v_beta] -> Gain3/1
  Gain3/1 -> Divide5/1
  [v_alpha] -> Divide6/2
  [i_alpha_ref] -> Add6/1
  [i_alpha_m] -> Add6/2
  [i_beta_ref] -> Add7/1
  Demux1/1 -> [i_alpha_m]
  Demux1/2 -> [i_beta_m]
  [i_beta_m] -> Add7/2
  Add6/1 -> [delta_i_alpha]
  Add7/1 -> [delta_i_beta]
  [delta_i_beta] -> Divide7/1
  [eta1] -> Divide7/2
  Divide7/1 -> Add10/3
  [delta_i_alpha] -> Divide8/1
  [eta2] -> Divide8/2
  Divide8/1 -> Add11/3
  Add10/1 -> Integrator/1
  Add11/1 -> Integrator1/1
  Gain5/1 -> Divide3/2
  Vref_LL/1 -> [vref]
  [vref] -> Magnitude Squared2/1
  [v_alpha] -> Divide9/2
  [v_beta] -> Divide10/1
  Divide5/1 -> Add10/1
  Divide9/1 -> Add10/2
  Divide6/1 -> Add11/1
  Divide10/1 -> Add11/2
  Ugabc/1 -> abc to Alpha-Beta-Zero1/1
  abc to Alpha-Beta-Zero1/1 -> Demux/1
  From38/1 -> ?
  [v_alpha] -> Add12/2
  From39/1 -> ?
  [v_beta] -> Add13/2
  Add12/1 -> [deltaV_alpha]
  Add13/1 -> [deltaV_beta]
  Divide11/1 -> Add10/4
  Divide12/1 -> Add11/4
  Gain4/1 -> Divide2/1
  Demux/1 -> [Ug_alpha]
  Demux/2 -> [Ug_beta]
  From26/1 -> Divide15/1, Divide13/1
  From/1 -> Divide15/2, Divide14/1
  From27/1 -> Divide16/1, Divide14/2
  Divide13/1 -> Add15/1
  Divide14/1 -> Add15/2
  Divide15/1 -> Add16/1
  Divide16/1 -> Add16/2
  Gain7/1 -> Divide17/1
  Gain8/1 -> Divide18/2
  From1/1 -> Divide18/1, Divide17/2
  Add15/1 -> Gain7/1
  Add16/1 -> Gain8/1
  Divide17/1 -> Goto19/1
  Divide18/1 -> Goto20/1
  From28/1 -> Divide19/1
  From29/1 -> Divide19/2
  From30/1 -> Divide20/1
  From31/1 -> Divide20/2
  Divide19/1 -> Add17/1
  Divide20/1 -> Add17/2
  Add17/1 -> Add18/1
  From32/1 -> Add18/2
  From33/1 -> Divide21/1
  From34/1 -> Divide21/2
  From35/1 -> Divide22/1
  From36/1 -> Divide22/2
  Divide21/1 -> Add19/1
  Divide22/1 -> Add19/2
  Add19/1 -> Add20/1
  From37/1 -> Add20/2
  Add18/1 -> Goto21/1
  Add20/1 -> Goto22/1
  [Ug_alpha] -> Add12/1
  [Ug_beta] -> Add13/1
  [mu] -> Divide4/1
  Step/1 -> Gamma_Slider/1
  Gamma_Slider/1 -> [Gamma]
  [Gamma] -> Divide11/2
  Divide4/1 -> [errorV]
  Add4/1 -> [omega_natural]
  [omega_natural] -> Divide6/1
  [errorV] -> Divide9/1
  Integrator/1 -> [v_alpha]
  [v_alpha] -> Gain6/1
  [Gamma] -> Divide12/1
  [deltaV_alpha] -> Divide11/1
  [deltaV_beta] -> Divide12/2
  [v_beta] -> Gain9/1
  Gain6/1 -> Inverse Clarke Transform/1
  Gain9/1 -> Inverse Clarke Transform/2
  Atan2/1 -> Goto27/1
  From53/1 -> Atan1/1
  From54/1 -> Atan1/2
  Atan1/1 -> Goto28/1
  fre_PLL/1 -> Gain4/1
  Sqrt/1 -> Vm/1  "Vm"
  Add2/1 -> [v2], Sqrt/1
  Magnitude Squared3/1 -> Add8/1
  [Ug_beta] -> Magnitude Squared3/1
  Magnitude Squared4/1 -> Add8/2
  [Ug_alpha] -> Magnitude Squared4/1
  Add8/1 -> Sqrt1/1
  Sqrt1/1 -> Um/1  "Um"
  Magnitude Squared5/1 -> Add9/1
  Sqrt2/1 -> Im/1  "Im"
  [i_beta_m] -> Magnitude Squared6/1
  Add9/1 -> Sqrt2/1
  [i_alpha_m] -> Magnitude Squared5/1
  Magnitude Squared6/1 -> Add9/2
  eps2_PV/1 -> [eps]
  eta2_PV/1 -> [eta2], [eta1]
  mu2_PV/1 -> [mu]

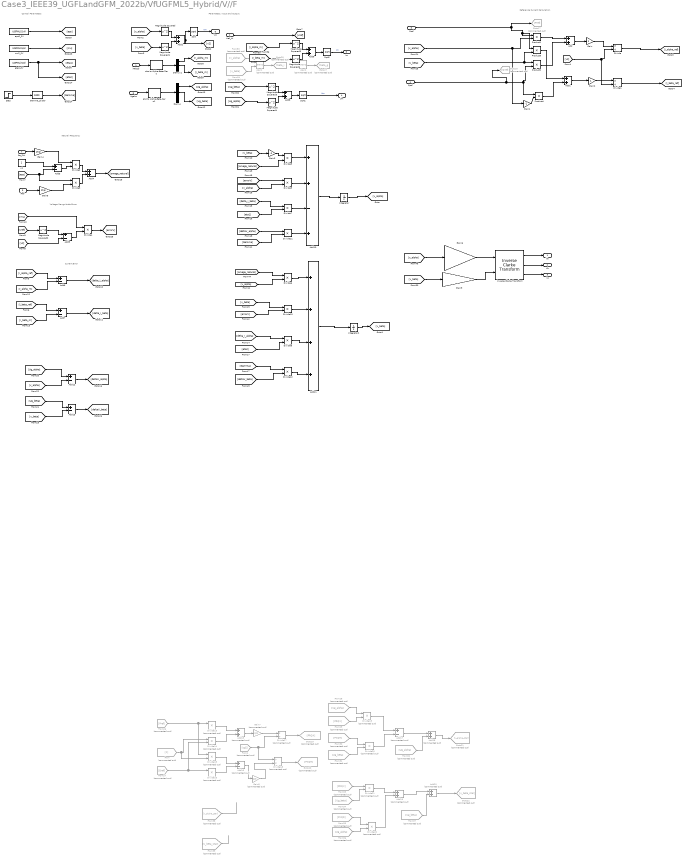
== system Case3_IEEE39_UGFLandGFM_2022b/VfUGFML5_Hybrid/V//F ==
  note: Natural Frequency
  note: Voltage Mangnitude Errror
  note: Current Error
  note: Control Parameters
  note: Parameters, Input and Output
  note: Reference Current Calculation
  iFabcb : Inport
  Vref_LL : Inport  Port=2
  Fref : Inport  Port=3
  Qref : Inport  Port=4
  Pref : Inport  Port=5
  Ugabc : Inport  Port=6
  fre_PLL : Inport  Port=7
  Add{,1..2,4,8..9} (6 alike) : Sum
  Add10 : Sum  Inputs=++-+
  Add11 : Sum  Inputs=++++
  Add{3,5..7,12..13} (6 alike) : Sum  Inputs=+-
  Add{15,18..20} (4 alike) : Sum  Commented=on
  Add16 : Sum  Commented=on  Inputs=+-
  Add17 : Sum  Commented=on  Inputs=+-
  Atan1 : Trigonometry  Commented=on  Operator=atan2
  Atan2 : Trigonometry  Commented=on  Operator=atan2
  Demux : Demux  Outputs=3
  Demux1 : Demux  Outputs=3
  Divide : Product  Inputs=*/
  Divide1 : Product  Inputs=*/
  Divide{2..12} (11 alike) : Product  Inputs=**
  Divide{13..16,19..22} (8 alike) : Product  Commented=on  Inputs=**
  Divide17 : Product  Commented=on  Inputs=*/
  Divide18 : Product  Commented=on  Inputs=/*
  From : From  Commented=on  GotoTag=X
  From1 : From  Commented=on  GotoTag=ug2
  From26 : From  Commented=on  GotoTag=Pref
  From27 : From  Commented=on  GotoTag=Qref
  From28 : From  Commented=on  GotoTag=Ug_alpha
  From29 : From  Commented=on  GotoTag=PRQX
  From30 : From  Commented=on  GotoTag=PXQR
  From31 : From  Commented=on  GotoTag=Ug_beta
  From32 : From  Commented=on  GotoTag=Ug_alpha
  From33 : From  Commented=on  GotoTag=PRQX
  From34 : From  Commented=on  GotoTag=Ug_beta
  From35 : From  Commented=on  GotoTag=PXQR
  From36 : From  Commented=on  GotoTag=Ug_alpha
  From37 : From  Commented=on  GotoTag=Ug_beta
  From38 : From  Commented=on  GotoTag=v_alpha_star
  From39 : From  Commented=on  GotoTag=v_beta_star
  From53 : From  Commented=on  GotoTag=v_alpha
  From54 : From  Commented=on  GotoTag=v_beta
  Gain : Gain
  Gain1 : Gain  Gain=-1
  Gain2 : Gain
  Gain3 : Gain  Gain=-1
  Gain4 : Gain  Gain=2*pi
  Gain5 : Gain  Gain=2*pi
  Gain6 : Gain  Gain=Vbase/sqrt(3)*sqrt(2)
  Gain7 : Gain  Commented=on  Gain=2/3
  Gain8 : Gain  Commented=on  Gain=2/3
  Gain9 : Gain  Gain=Vbase/sqrt(3)*sqrt(2)
  Gamma_Slider : simulink/Math Operations/Slider Gain  gain=1000  low=0  high=1000
  Goto17 : Goto  Commented=on  GotoTag=Pref
  Goto18 : Goto  Commented=on  GotoTag=Qref
  Goto19 : Goto  Commented=on  GotoTag=PRQX
  Goto20 : Goto  Commented=on  GotoTag=PXQR
  Goto21 : Goto  Commented=on  GotoTag=v_alpha_star
  Goto22 : Goto  Commented=on  GotoTag=v_beta_star
  Goto27 : Goto  Commented=on  GotoTag=theta_g  TagVisibility=global
  Goto28 : Goto  Commented=on  GotoTag=theta_i  TagVisibility=global
  Integrator : Integrator  InitialCondition=1  LimitOutput=on  UpperSaturationLimit=2  LowerSaturationLimit=-2  ZeroCross=off
  Integrator1 : Integrator  InitialCondition=0.0001  LimitOutput=on  UpperSaturationLimit=2  LowerSaturationLimit=-2  ZeroCross=off
  Inverse Clarke Transform : mcbcontrolslib/Inverse Clarke Transform  PhaseInput=Two inputs  EnPowerInv=off
      settings: LibrarySourceBlock=mcblib/Controls/Math Transforms/Inverse Clarke Transform
  Magnitude Squared{,1..6} (7 alike) : Math  Operator=square
  Product{1..4} (4 alike) : Product
  Sqrt : Sqrt
  Sqrt1 : Sqrt
  Sqrt2 : Sqrt
  Step : Step  Time=0.1  Before=1  After=0  SampleTime=0
  abc to Alpha-Beta-Zero : spsabctoAlphaBetaZeroLib/abc to Alpha-Beta-Zero
  abc to Alpha-Beta-Zero1 : spsabctoAlphaBetaZeroLib/abc to Alpha-Beta-Zero
  eps2_PV : Constant  Value=UGFML(5,4)
  eta2_PV : Constant  Value=UGFML(5,6)
  mu2_PV : Constant  Value=UGFML(5,5)
  u1 : Constant
  Va : Outport
  Vb : Outport  Port=2
  Vc : Outport  Port=3
  Um : Outport  Port=4
  Im : Outport  Port=5
  Vm : Outport  Port=6
  wires:
  iFabcb/1 -> abc to Alpha-Beta-Zero/1
  Inverse Clarke Transform/1 -> Va/1
  Inverse Clarke Transform/2 -> Vb/1
  Inverse Clarke Transform/3 -> Vc/1
  abc to Alpha-Beta-Zero/1 -> Demux1/1
  Integrator1/1 -> [v_beta]
  Pref/1 -> Product3/1, Product1/1, Goto17/1
  [v_alpha] -> Gain1/1, Product1/2
  [v_beta] -> Product3/2, Product2/1
  Qref/1 -> Goto18/1, Product2/2, Product4/1
  Product1/1 -> Add/1
  Product2/1 -> Add/2
  Gain1/1 -> Product4/2
  Product3/1 -> Add1/1
  Product4/1 -> Add1/2
  Add/1 -> Gain/1
  Add1/1 -> Gain2/1
  [v_alpha] -> Magnitude Squared/1
  [v_beta] -> Magnitude Squared1/1
  Magnitude Squared/1 -> Add2/1
  Magnitude Squared1/1 -> Add2/2
  Gain/1 -> Divide/1
  [v2] -> Divide/2, Divide1/2
  Gain2/1 -> Divide1/1
  Divide/1 -> [i_alpha_ref]
  Divide1/1 -> [i_beta_ref]
  u1/1 -> Add3/1
  [eps] -> Divide3/1, Add3/2
  Add3/1 -> Divide2/2
  Fref/1 -> Gain5/1
  Divide2/1 -> Add4/1
  Divide3/1 -> Add4/2
  [v2] -> Add5/2
  Magnitude Squared2/1 -> Add5/1
  Add5/1 -> Divide4/2
  [errorV] -> Divide10/2
  [omega_natural] -> Divide5/2
  [v_beta] -> Gain3/1
  Gain3/1 -> Divide5/1
  [v_alpha] -> Divide6/2
  [i_alpha_ref] -> Add6/1
  [i_alpha_m] -> Add6/2
  [i_beta_ref] -> Add7/1
  Demux1/1 -> [i_alpha_m]
  Demux1/2 -> [i_beta_m]
  [i_beta_m] -> Add7/2
  Add6/1 -> [delta_i_alpha]
  Add7/1 -> [delta_i_beta]
  [delta_i_beta] -> Divide7/1
  [eta1] -> Divide7/2
  Divide7/1 -> Add10/3
  [delta_i_alpha] -> Divide8/1
  [eta2] -> Divide8/2
  Divide8/1 -> Add11/3
  Add10/1 -> Integrator/1
  Add11/1 -> Integrator1/1
  Gain5/1 -> Divide3/2
  Vref_LL/1 -> [vref]
  [vref] -> Magnitude Squared2/1
  [v_alpha] -> Divide9/2
  [v_beta] -> Divide10/1
  Divide5/1 -> Add10/1
  Divide9/1 -> Add10/2
  Divide6/1 -> Add11/1
  Divide10/1 -> Add11/2
  Ugabc/1 -> abc to Alpha-Beta-Zero1/1
  abc to Alpha-Beta-Zero1/1 -> Demux/1
  From38/1 -> ?
  [v_alpha] -> Add12/2
  From39/1 -> ?
  [v_beta] -> Add13/2
  Add12/1 -> [deltaV_alpha]
  Add13/1 -> [deltaV_beta]
  Divide11/1 -> Add10/4
  Divide12/1 -> Add11/4
  Gain4/1 -> Divide2/1
  Demux/1 -> [Ug_alpha]
  Demux/2 -> [Ug_beta]
  From26/1 -> Divide15/1, Divide13/1
  From/1 -> Divide15/2, Divide14/1
  From27/1 -> Divide16/1, Divide14/2
  Divide13/1 -> Add15/1
  Divide14/1 -> Add15/2
  Divide15/1 -> Add16/1
  Divide16/1 -> Add16/2
  Gain7/1 -> Divide17/1
  Gain8/1 -> Divide18/2
  From1/1 -> Divide18/1, Divide17/2
  Add15/1 -> Gain7/1
  Add16/1 -> Gain8/1
  Divide17/1 -> Goto19/1
  Divide18/1 -> Goto20/1
  From28/1 -> Divide19/1
  From29/1 -> Divide19/2
  From30/1 -> Divide20/1
  From31/1 -> Divide20/2
  Divide19/1 -> Add17/1
  Divide20/1 -> Add17/2
  Add17/1 -> Add18/1
  From32/1 -> Add18/2
  From33/1 -> Divide21/1
  From34/1 -> Divide21/2
  From35/1 -> Divide22/1
  From36/1 -> Divide22/2
  Divide21/1 -> Add19/1
  Divide22/1 -> Add19/2
  Add19/1 -> Add20/1
  From37/1 -> Add20/2
  Add18/1 -> Goto21/1
  Add20/1 -> Goto22/1
  [Ug_alpha] -> Add12/1
  [Ug_beta] -> Add13/1
  [mu] -> Divide4/1
  Step/1 -> Gamma_Slider/1
  Gamma_Slider/1 -> [Gamma]
  [Gamma] -> Divide11/2
  Divide4/1 -> [errorV]
  Add4/1 -> [omega_natural]
  [omega_natural] -> Divide6/1
  [errorV] -> Divide9/1
  Integrator/1 -> [v_alpha]
  [v_alpha] -> Gain6/1
  [Gamma] -> Divide12/1
  [deltaV_alpha] -> Divide11/1
  [deltaV_beta] -> Divide12/2
  [v_beta] -> Gain9/1
  Gain6/1 -> Inverse Clarke Transform/1
  Gain9/1 -> Inverse Clarke Transform/2
  Atan2/1 -> Goto27/1
  From53/1 -> Atan1/1
  From54/1 -> Atan1/2
  Atan1/1 -> Goto28/1
  fre_PLL/1 -> Gain4/1
  Sqrt/1 -> Vm/1  "Vm"
  Add2/1 -> [v2], Sqrt/1
  Magnitude Squared3/1 -> Add8/1
  [Ug_beta] -> Magnitude Squared3/1
  Magnitude Squared4/1 -> Add8/2
  [Ug_alpha] -> Magnitude Squared4/1
  Add8/1 -> Sqrt1/1
  Sqrt1/1 -> Um/1  "Um"
  Magnitude Squared5/1 -> Add9/1
  Sqrt2/1 -> Im/1  "Im"
  [i_beta_m] -> Magnitude Squared6/1
  Add9/1 -> Sqrt2/1
  [i_alpha_m] -> Magnitude Squared5/1
  Magnitude Squared6/1 -> Add9/2
  eps2_PV/1 -> [eps]
  eta2_PV/1 -> [eta2], [eta1]
  mu2_PV/1 -> [mu]

== system Case3_IEEE39_UGFLandGFM_2022b/G3_GFL/PV_PQ3/Freq_Droop ==
  Pref : Inport
  Fref : Inport  Port=2
  Freq : Inport  Port=3
  D : Inport  Port=4
  Divide : Product  Inputs=*/
  Product : Product
  Product1 : Product
  S_base : Constant  Value=Sbase
  Saturation : Saturate  UpperLimit=10*Sbase  LowerLimit=0  ZeroCross=off
  Sum : Sum  Inputs=|+-
  Sum1 : Sum  Inputs=|+-
  Transfer Fcn : TransferFcn  Denominator=[0.318 1]
  Pset : Outport
  wires:
  Freq/1 -> Sum/1
  Fref/1 -> Sum/2, Divide/2
  S_base/1 -> Product/2
  D/1 -> Product1/1
  Product/1 -> Product1/2
  Pref/1 -> Sum1/1
  Product1/1 -> Sum1/2
  Saturation/1 -> Pset/1
  Sum1/1 -> Saturation/1
  Sum/1 -> Divide/1
  Transfer Fcn/1 -> Product/1
  Divide/1 -> Transfer Fcn/1

== system Case3_IEEE39_UGFLandGFM_2022b/G3_GFL/PV_PQ3/Subsystem2 ==
  note: Iq_ref
  note: Id
  note: Id_ref
  note: Ud
  note: Uq
  note: eq
  note: ed
  note: Ioq
  note: Id
  Vabcp : Inport
  Iabcp : Inport  Port=2
  IFabcp : Inport  Port=3
  P_set : Inport  Port=4
  Q_set : Inport  Port=5
  L1 : Inport  Port=6
  Add : Sum  Inputs=++-
  Add1 : Sum  Inputs=+++
  Demux{,1..3} (4 alike) : Demux  Outputs=3
  Discrete Transfer Fcn1 : DiscreteTransferFcn  Numerator=[0.2 0]  Denominator=[1 -0.8]  InitialStates=[1 1 1]  SampleTime=5e-4
  Discrete Transfer Fcn3 : DiscreteTransferFcn  Numerator=[0.2 0]  Denominator=[1 -0.8]  SampleTime=5e-4
  Discrete Transfer Fcn4 : DiscreteTransferFcn  Numerator=[0.2 0]  Denominator=[1 -0.8]  SampleTime=5e-4
  Mux : Mux  Inputs=3
  PID Controller1 : slpidlib/PID Controller  Controller=PI  Form=Parallel  TimeDomain=Discrete-time  UseExternalTs=off  SampleTime=5e-4  IntegratorMethod=Forward Euler  FilterMethod=Forward Euler  ControllerParametersSource=internal  P=188.4  I=4000  UseKiTs=off  D=0  N=100  UseFilter=on  TunerSelectOption=Transfer Function Based (PID Tuner App)  InitialConditionSource=internal  InitialConditionForIntegrator=0  InitialConditionForFilter=0  DifferentiatorICPrevScaledInput=0  ExternalReset=none  TrackingMode=off  Kt=1  LimitOutput=off  SatLimitsSource=internal  UpperSaturationLimit=inf  LowerSaturationLimit=-inf  LinearizeAsGain=on  AntiWindupMode=none  Kb=1  LimitIntegrator=off  UpperIntegratorSaturationLimit=inf  LowerIntegratorSaturationLimit=-inf  POutMin=[]  POutMax=[]  IOutMin=[]  IOutMax=[]  DOutMin=[]  DOutMax=[]  NOutMin=[]  NOutMax=[]  SumOutMin=[]  SumOutMax=[]  SaturationOutMin=[]  SaturationOutMax=[]  PParamMin=[]  PParamMax=[]  IParamMin=[]  IParamMax=[]  DParamMin=[]  DParamMax=[]  NParamMin=[]  NParamMax=[]  KbParamMin=[]  KbParamMax=[]  KtParamMin=[]  KtParamMax=[]  KbOutMin=[]  KbOutMax=[]  KtOutMin=[]  KtOutMax=[]  IntegratorOutMin=[]  IntegratorOutMax=[]  FilterOutMin=[]  FilterOutMax=[]  SumI1OutMin=[]  SumI1OutMax=[]  SumI2OutMin=[]  SumI2OutMax=[]  SumI3OutMin=[]  SumI3OutMax=[]  SumI4OutMin=[]  SumI4OutMax=[]  SumDOutMin=[]  SumDOutMax=[]  DifferentiatorOutMin=[]  DifferentiatorOutMax=[]  FilterDiffOutCoefMin=[]  FilterDiffOutCoefMax=[]  ReciprocalOutMin=[]  ReciprocalOutMax=[]  SumDenOutMin=[]  SumDenOutMax=[]  SumNumOutMin=[]  SumNumOutMax=[]  DivideOutMin=[]  DivideOutMax=[]  UdiffTsProdOutMin=[]  UdiffTsProdOutMax=[]  NTsProdOutMin=[]  NTsProdOutMax=[]  UintegralTsProdOutMin=[]  UintegralTsProdOutMax=[]  UngainTsProdOutMin=[]  UngainTsProdOutMax=[]  IntegratorContinuousStateAttributes=''  IntegratorStateMustResolveToSignalObject=off  IntegratorRTWStateStorageClass=Auto  FilterContinuousStateAttributes=''  FilterStateMustResolveToSignalObject=off  FilterRTWStateStorageClass=Auto  ParallelPVariant=InternalParameters  IdealPVariant=Disabled  IVariant=InternalParameters  DVariant=Disabled  IntegratorVariant=Discrete  SatVariant=Disabled  AWVariant=Passthrough  PCopyVariant=Disabled  TRVariant=Disabled  FdbkBlocksVariant=Forward  IdealPFdbkVariant=Disabled  SatFdbkVariant=Disabled  DerivativeFilterVariant=Disabled  NVariant=Disabled  NCopyVariant=Disabled_SignalSpec  FilterICVariant=Disabled  IntegratorICVariant=InternalICs  ExternalResetVariant=Disabled  TRSumVariant=Passthrough  SumFdbkVariant=Disabled  SumVariant=Sum_PI  TsampFilterVariant=InternalTs  TsampNgainVariant=Passthrough  TsampIntegralVariant=Disabled_SignalSpec  ExternalSaturationOutDataTypeStr=Inherit: Same as second input
  PID Controller2 : slpidlib/PID Controller  Controller=PI  Form=Parallel  TimeDomain=Discrete-time  UseExternalTs=off  SampleTime=5e-4  IntegratorMethod=Forward Euler  FilterMethod=Forward Euler  ControllerParametersSource=internal  P=188.4  I=4000  UseKiTs=off  D=0  N=100  UseFilter=on  TunerSelectOption=Transfer Function Based (PID Tuner App)  InitialConditionSource=internal  InitialConditionForIntegrator=0  InitialConditionForFilter=0  DifferentiatorICPrevScaledInput=0  ExternalReset=none  TrackingMode=off  Kt=1  LimitOutput=off  SatLimitsSource=internal  UpperSaturationLimit=inf  LowerSaturationLimit=-inf  LinearizeAsGain=on  AntiWindupMode=none  Kb=1  LimitIntegrator=off  UpperIntegratorSaturationLimit=inf  LowerIntegratorSaturationLimit=-inf  POutMin=[]  POutMax=[]  IOutMin=[]  IOutMax=[]  DOutMin=[]  DOutMax=[]  NOutMin=[]  NOutMax=[]  SumOutMin=[]  SumOutMax=[]  SaturationOutMin=[]  SaturationOutMax=[]  PParamMin=[]  PParamMax=[]  IParamMin=[]  IParamMax=[]  DParamMin=[]  DParamMax=[]  NParamMin=[]  NParamMax=[]  KbParamMin=[]  KbParamMax=[]  KtParamMin=[]  KtParamMax=[]  KbOutMin=[]  KbOutMax=[]  KtOutMin=[]  KtOutMax=[]  IntegratorOutMin=[]  IntegratorOutMax=[]  FilterOutMin=[]  FilterOutMax=[]  SumI1OutMin=[]  SumI1OutMax=[]  SumI2OutMin=[]  SumI2OutMax=[]  SumI3OutMin=[]  SumI3OutMax=[]  SumI4OutMin=[]  SumI4OutMax=[]  SumDOutMin=[]  SumDOutMax=[]  DifferentiatorOutMin=[]  DifferentiatorOutMax=[]  FilterDiffOutCoefMin=[]  FilterDiffOutCoefMax=[]  ReciprocalOutMin=[]  ReciprocalOutMax=[]  SumDenOutMin=[]  SumDenOutMax=[]  SumNumOutMin=[]  SumNumOutMax=[]  DivideOutMin=[]  DivideOutMax=[]  UdiffTsProdOutMin=[]  UdiffTsProdOutMax=[]  NTsProdOutMin=[]  NTsProdOutMax=[]  UintegralTsProdOutMin=[]  UintegralTsProdOutMax=[]  UngainTsProdOutMin=[]  UngainTsProdOutMax=[]  IntegratorContinuousStateAttributes=''  IntegratorStateMustResolveToSignalObject=off  IntegratorRTWStateStorageClass=Auto  FilterContinuousStateAttributes=''  FilterStateMustResolveToSignalObject=off  FilterRTWStateStorageClass=Auto  ParallelPVariant=InternalParameters  IdealPVariant=Disabled  IVariant=InternalParameters  DVariant=Disabled  IntegratorVariant=Discrete  SatVariant=Disabled  AWVariant=Passthrough  PCopyVariant=Disabled  TRVariant=Disabled  FdbkBlocksVariant=Forward  IdealPFdbkVariant=Disabled  SatFdbkVariant=Disabled  DerivativeFilterVariant=Disabled  NVariant=Disabled  NCopyVariant=Disabled_SignalSpec  FilterICVariant=Disabled  IntegratorICVariant=InternalICs  ExternalResetVariant=Disabled  TRSumVariant=Passthrough  SumFdbkVariant=Disabled  SumVariant=Sum_PI  TsampFilterVariant=InternalTs  TsampNgainVariant=Passthrough  TsampIntegralVariant=Disabled_SignalSpec  ExternalSaturationOutDataTypeStr=Inherit: Same as second input
  PLL (3ph) : spsPLL3phLib/PLL (3ph)  Fmin=59.5  Par_Init=[0, 60]  ParK=[180, 3200, 1]  TcD=1e-4  MaxRateChangeFreq=12  FilterCutOffFreq=25  Ts=1e-5  AGC=on
  Subsystem1 : Subsystem
  Sum1 : Sum  Inputs=|+-
  Sum2 : Sum  Inputs=|+-
  Terminator{,1..4} (5 alike) : Terminator
  WL : Subsystem
  WL1 : Subsystem
  abc to dq0 : spsabctodq0Lib/abc to dq0  Alignment=90 degrees behind phase A axis
  abc to dq1 : spsabctodq0Lib/abc to dq0  Alignment=90 degrees behind phase A axis
  abc to dq2 : spsabctodq0Lib/abc to dq0  Alignment=90 degrees behind phase A axis
  constant : Constant  Value=0
  dq0 to abc : spsdq0toabcLib/dq0 to abc  Alignment=90 degrees behind phase A axis
  Va : Outport  VectorParamsAs1DForOutWhenUnconnected=off
  Vb : Outport  Port=2  VectorParamsAs1DForOutWhenUnconnected=off
  Vc : Outport  Port=3  VectorParamsAs1DForOutWhenUnconnected=off
  wires:
  abc to dq0/1 -> Discrete Transfer Fcn3/1
  PLL (3ph)/2 -> [wt], abc to dq1/2, abc to dq2/2, abc to dq0/2
  Demux1/1 -> Add/1, Subsystem1/3(Ud)
  L1/1 -> WL/3(L), WL1/3(L)
  WL/1(Out1) -> Add/3
  [freq] -> WL1/2(freq), WL/2(freq)
  PLL (3ph)/1 -> [freq]
  Demux2/1 -> Va/1
  Add/1 -> Mux/1
  PID Controller2/1 -> Add1/2
  Demux2/2 -> Vb/1
  WL1/1(Out1) -> Add1/3
  Demux1/2 -> Add1/1
  Add1/1 -> Mux/2
  Mux/1 -> dq0 to abc/1
  Demux2/3 -> Vc/1
  dq0 to abc/1 -> Demux2/1
  Subsystem1/1(Id_ref) -> Sum1/1
  PID Controller1/1 -> Add/2
  [wt] -> dq0 to abc/2
  Subsystem1/2(Iq_ref) -> Sum2/1
  Demux1/3 -> Terminator/1
  Demux/3 -> Terminator1/1
  constant/1 -> Mux/3
  IFabcp/1 -> abc to dq2/1
  abc to dq2/1 -> Discrete Transfer Fcn4/1
  Demux3/3 -> Terminator2/1
  Demux3/2 -> Sum2/2, WL/1(In1)
  Demux3/1 -> Sum1/2, WL1/1(In1)
  Sum1/1 -> PID Controller1/1
  Sum2/1 -> PID Controller2/1
  P_set/1 -> Subsystem1/1(P_ref)
  Q_set/1 -> Subsystem1/2(Q_ref)
  Discrete Transfer Fcn3/1 -> Demux/1
  Discrete Transfer Fcn4/1 -> Demux3/1
  Demux/1 -> Terminator3/1
  Demux/2 -> Terminator4/1
  Discrete Transfer Fcn1/1 -> Demux1/1
  Iabcp/1 -> abc to dq0/1
  Vabcp/1 -> abc to dq1/1, PLL (3ph)/1
  abc to dq1/1 -> Discrete Transfer Fcn1/1

== system Case3_IEEE39_UGFLandGFM_2022b/GFM4/PV_PQ3/Freq_Droop ==
  Pref : Inport
  Fref : Inport  Port=2
  Pmeans : Inport  Port=3
  Add : Sum  Inputs=+-
  Add1 : Sum
  Divide : Product  Inputs=*/
  Product : Product
  S_base : Constant  Value=Sbase
  Saturation : Saturate  UpperLimit=2  LowerLimit=-2  ZeroCross=off
  Transfer Fcn2 : TransferFcn  Denominator=[2*IBR(2,5) IBR(2,4)]
  fset : Outport
  wires:
  Pref/1 -> Add/1
  Pmeans/1 -> Add/2
  S_base/1 -> Divide/2
  Transfer Fcn2/1 -> Product/1
  Add1/1 -> fset/1
  Saturation/1 -> Add1/1
  Product/1 -> Saturation/1
  Add/1 -> Divide/1
  Fref/1 -> Add1/2, Product/2
  Divide/1 -> Transfer Fcn2/1
